simulink model "UPE_max_final"  (Simulink 7.9)
settings: Solver=ode3  StartTime=0.0  StopTime=0.05  FixedStep=1e-10  RelTol=1e-3
settings Model: Creator=kacka  LastModifiedBy=kacka
settings SolverCC: AlgebraicLoopSolver=LineSearch
settings DataIOCC: Decimation=10000  LimitDataPoints=off

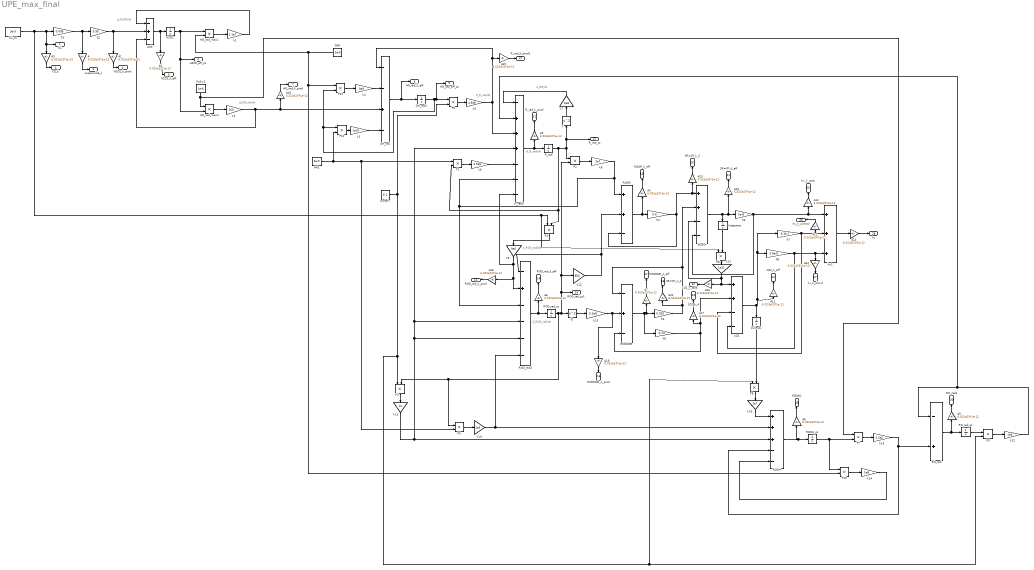
== system UPE_max_final ==
  note: d_H2O2/dt
  note: d_R_rad/dt
  note: d_R_rad/dt
  note: d_ROO_rad/dt
  note: d_RR/dt
  note: d_ROO_rad/dt
  note: d_HO_rad/dt
  1O2 : Sum  Inputs=++--
  1O2_ss1 : Integrator  LowerSaturationLimit=0
  3R=O* : Sum  Inputs=++--
  A{,1..13,15..24} (24 alike) : Gain  Gain=6.022e23*1e-12
  AH1 : Constant  Value=3e-5
  Add : Sum  Inputs=-+-
  Fe2+2 : Constant  Value=1e-6
  GSH : Constant  Value=1e-6
  H2O2 : Integrator
  HO_rad_max1 : Product  RndMeth=Zero
  HO_rad_max2 : Product  RndMeth=Zero
  Integrator : Integrator
  O2_ss : Constant  Value=3e-5
  OH_rad : Sum  Inputs=--+-
  OH_rad1 : Integrator  LowerSaturationLimit=0
  P{0..12} (13 alike) : Product  RndMeth=Zero
  ROOH : Sum  Inputs=+++--
  ROOH_ss : Integrator  LowerSaturationLimit=0
  ROOOOR : Sum  Inputs=-+-
  ROOR : Sum  Inputs=++-
  ROO_rad2 : Sum  Inputs=-+----
  ROO_rad_ss : Integrator  LowerSaturationLimit=0
  RO_rad : Sum  Inputs=-+
  RO_rad_ss : Integrator  LowerSaturationLimit=0
  R_rad : Integrator  LowerSaturationLimit=0
  R_rad5 : Sum  Inputs=-+++---
  f : Math  Operator=square  SaturateOnIntegerOverflow=on
  f2 : Math  Operator=square  SaturateOnIntegerOverflow=on
  fi1 : Gain  Gain=0.008
  fi2 : Gain  Gain=0.95
  fi3 : Gain  Gain=0.6
  fi4 : Gain  Gain=0.025
  fi5 : Gain  Gain=0.14
  fi6 : Gain  Gain=1e-8
  fi7 : Gain  Gain=9.3e-7
  fi8 : Gain  Gain=3.9e-6
  hv1 : Sum  Inputs=+++
  k1 : Gain  Gain=2.1e7
  k10 : Gain  Gain=1e5
  k11 : Gain  Gain=10
  k12 : Gain  Gain=800
  k13 : Gain  Gain=3.2e8
  k14 : Gain  Gain=1e8
  k15 : Gain  Gain=3.2e2
  k16 : Gain  Gain=1e7
  k17 : Gain  Gain=1e11
  k2 : Gain  Gain=100
  k22 : Gain  Gain=1e6
  k3 : Gain  Gain=1e10
  k4 : Gain  Gain=9e9
  k5 : Gain  Gain=4.6e8
  k6 : Gain  Gain=4.5e6
  k7 : Gain  Gain=2e8
  k8 : Gain  Gain=5e7
  k9 : Gain  Gain=9e6
  protein : Constant  Value=6.1
  O2 : Outport
  O2_k : Outport  Port=2
  superoxide_k : Outport  Port=3
  H2O2_k_prod : Outport  Port=4
  H2O2_k_eff : Outport  Port=5
  H2O2_eff_ss : Outport  Port=6
  HO_rad_k_prod : Outport  Port=7
  HO_rad_k_eff : Outport  Port=8
  HO_rad_eff_ss : Outport  Port=9
  R_rad_k_prod1 : Outport  Port=10
  R_rad_k_prod : Outport  Port=11
  R_rad_ss : Outport  Port=12
  ROO_rad_k_prod : Outport  Port=13
  ROO_rad_k_eff : Outport  Port=14
  ROO_rad_ss1 : Outport  Port=15
  ROOOOR_k_prod : Outport  Port=16
  ROOOOR_k_eff : Outport  Port=17
  3R=O*_k_4 : Outport  Port=18
  ROOR_k_eff : Outport  Port=19
  3R=O*_k_2 : Outport  Port=20
  3R=O*_k_eff : Outport  Port=21
  1O2_k_carb : Outport  Port=22
  1O2_k_4 : Outport  Port=23
  1O2_k_eff : Outport  Port=24
  hv_k_carb : Outport  Port=25
  hv_k_unimol : Outport  Port=26
  hv_k_dimol : Outport  Port=27
  hv : Outport  Port=28
  ROOH1 : Outport  Port=29
  RO_rad1 : Outport  Port=30
  wires:
  O2_ss/1 -> fi1/1, A3/1, O2/1, P3/1, P6/1
  fi1/1 -> fi2/1, A/1
  fi2/1 -> Add/2, A1/1
  A/1 -> superoxide_k/1
  A1/1 -> H2O2_k_prod/1
  A3/1 -> O2_k/1
  P0/1 -> k5/1
  protein/1 -> P4/1, P9/2, P8/1, P0/2
  R_rad5/1 -> R_rad/1, A5/1
  P1/1 -> k6/1
  P2/1 -> k8/1
  P3/1 -> k9/1
  ROOR/1 -> fi3/1, A2/1
  ROOOOR/1 -> fi5/1, fi4/1, A7/1
  fi3/1 -> ROOR/3, 3R=O*/1, A23/1
  fi4/1 -> ROOOOR/1, 3R=O*/2, A24/1
  hv1/1 -> A13/1
  A13/1 -> hv/1
  3R=O*/1 -> fi6/1, A10/1, Integrator/1
  fi6/1 -> 3R=O*/4, hv1/1, A12/1
  fi7/1 -> 1O2/3, hv1/2, A21/1
  fi8/1 -> 1O2/4, hv1/3, A22/1
  1O2/1 -> 1O2_ss1/1, fi7/1, fi8/1, A11/1
  k17/1 -> 3R=O*/3, 1O2/1, A20/1
  P6/1 -> k17/1
  Integrator/1 -> P6/2
  fi5/1 -> 1O2/2, A17/1, ROOOOR/3
  f2/1 -> k13/1
  k13/1 -> ROOOOR/2, A19/1
  k15/1 -> ROOH/4, RO_rad/2
  P7/1 -> k15/1
  ROOH_ss/1 -> P7/2, P10/1
  ROOH/1 -> ROOH_ss/1, A8/1
  k16/1 -> ROOH/1
  P8/1 -> k16/1
  1O2_ss1/1 -> P8/2
  RO_rad/1 -> RO_rad_ss/1, A9/1
  ROO_rad_ss/1 -> f2/1, P2/2, k12/1, ROO_rad_ss1/1, P4/2, P5/1
  ROO_rad2/1 -> ROO_rad_ss/1, A6/1
  R_rad/1 -> P2/1, f/1, R_rad_ss/1, P3/2, P1/2
  k8/1 -> ROOR/1, ROO_rad2/3, R_rad5/6
  k12/1 -> ROO_rad2/1, ROOR/2
  k5/1 -> R_rad5/3, OH_rad/1, A15/1
  f/1 -> k7/1
  k7/1 -> R_rad5/1
  P5/1 -> k10/1
  P4/1 -> k11/1
  k11/1 -> ROOH/3, ROO_rad2/4, R_rad5/4, ROO_rad2/5
  k9/1 -> R_rad5/7, ROO_rad2/2, A18/1
  k10/1 -> ROOH/2, ROO_rad2/6
  RO_rad_ss/1 -> P9/1
  P9/1 -> k22/1
  k22/1 -> R_rad5/2, RO_rad/1
  AH1/1 -> P1/1, P5/2, P12/2
  A5/1 -> R_rad_k_prod/1
  A6/1 -> ROO_rad_k_eff/1
  A2/1 -> ROOR_k_eff/1
  A7/1 -> ROOOOR_k_eff/1
  A8/1 -> ROOH1/1
  A9/1 -> RO_rad1/1
  A10/1 -> 3R=O*_k_eff/1
  A11/1 -> 1O2_k_eff/1
  A12/1 -> hv_k_carb/1
  A15/1 -> R_rad_k_prod1/1
  k6/1 -> R_rad5/5
  k1/1 -> Add/1
  Add/1 -> H2O2/1, A4/1
  GSH/1 -> HO_rad_max1/2, P10/2, P11/1
  HO_rad_max1/1 -> k1/1
  H2O2/1 -> HO_rad_max1/1, HO_rad_max2/2, H2O2_eff_ss/1
  A16/1 -> HO_rad_k_prod/1
  HO_rad_max2/1 -> k2/1
  k2/1 -> OH_rad/3, A16/1, Add/3
  A4/1 -> H2O2_k_eff/1
  P10/1 -> k14/1
  k14/1 -> ROOH/5
  Fe2+2/1 -> HO_rad_max2/1, P7/1
  P11/1 -> k4/1
  k4/1 -> OH_rad/2
  P12/1 -> k3/1
  k3/1 -> OH_rad/4
  OH_rad1/1 -> P0/1, HO_rad_eff_ss/1, P12/1, P11/2
  OH_rad/1 -> OH_rad1/1, HO_rad_k_eff/1
  A18/1 -> ROO_rad_k_prod/1
  A19/1 -> ROOOOR_k_prod/1
  A17/1 -> 1O2_k_4/1
  A20/1 -> 1O2_k_carb/1
  A21/1 -> hv_k_unimol/1
  A22/1 -> hv_k_dimol/1
  A23/1 -> 3R=O*_k_2/1
  A24/1 -> 3R=O*_k_4/1
